simulink model "automata"  (R2020b)
settings: Solver=FixedStepAuto  StartTime=0.0  StopTime=inf  FixedStep=2e-2  RelTol=1e-3
libraries: simulink x3
settings Model: Creator=GoniR  LastModifiedBy=GoniR

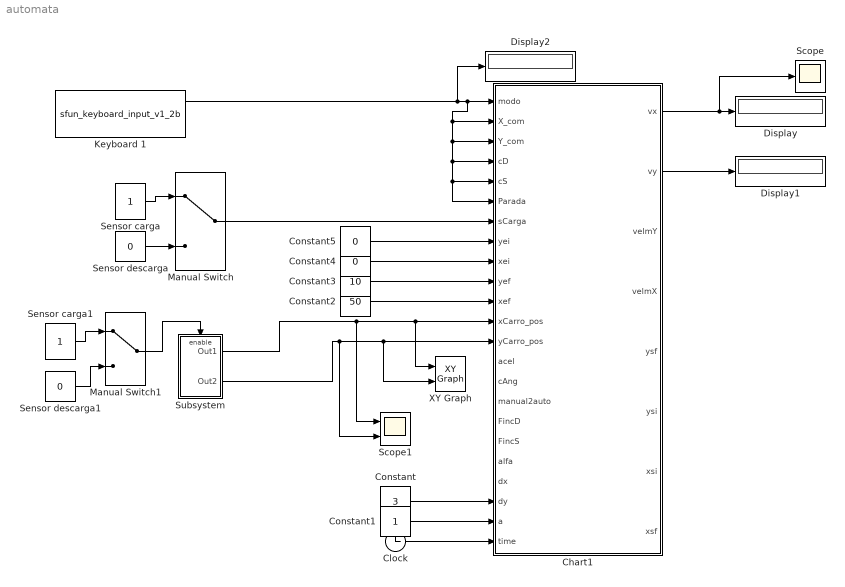
== system automata ==
  Chart1 : Stateflow chart  TreatAsAtomicUnit=on
      settings: PortSchema="{\"entries\":[{\"content\":{\"sides\":[{\"content\":{\"connectorIds\":[\"In5\",\"In1\",\"In2\",\"In12\",\"In13\",\"In18\",\"In14\",\"In9\",\"In10\",\"In4\",\"In11\",\"In16\",\"In22\",\"In23\",\"In15\",\"In3\",\"In17\",\"In19\",\"In7\",\"In8\",\"In6\",\"In21\",\"In20\"]},\"type\":\"ConnectorPlacement.EquallySpacedRectSide\",\"uuid\":\"1e4dd542-1771-4859-b91f-fc1cb250280a\"},{\"content\":{\"connectorIds\":[\"Out1\",\"Out2\",\"Out3\",\"Out4\",\"Out5\",\"Out6\",\"Out7\",\"Out8\"],\"side\":\"RIGHT\"},\"type\":\"ConnectorPlacement.EquallySpacedRectSide\",\"uuid\":\"bb5e6521-c449-4a1c-9147-094c14f63665\"},{\"content\":{\"connectorIds\":[],\"side\":\"TOP\"},\"type\":\"ConnectorPlacement.EquallySpacedRectSide\",\"uuid\":\"54352a45-add1-4eb7-bb1e-2f57d731739f\"},{\"content\":{\"connectorIds\":[],\"side\":\"HIDDEN\"},\"type\":\"ConnectorPlacement.EquallySpacedRectSide\",\"uuid\":\"3e291a91-093a-4ab5-80ab-be4d5a353953\"}]},\"type\":\"ConnectorPlacement.EquallySpacedConnector\",\"uuid\":\"db8c49e8-a9b8-459f-b7fa-0d865c8e3061\"}],\"packageUris\":[\"http://schema.mathworks.com/mf0/Connector/R2020b\"],\"version\":\"1.0\"}"
  Clock : Clock
  Constant : Constant  Value=3
  Constant1 : Constant
  Constant2 : Constant  Value=50
  Constant3 : Constant  Value=10
  Constant4 : Constant  Value=0
  Constant5 : Constant  Value=0
  Display : Display
  Display1 : Display
  Display2 : Display
  Keyboard 1 : M-S-Function  FunctionName=sfun_keyboard_input_v1_2b  mask(Keyboard Input){}
      mask help: Keyboard Input
      mask Display: fprintf('Keyboard');
  Manual Switch : ManualSwitch
  Manual Switch1 : ManualSwitch
  Scope : Scope
  Scope1 : Scope  NumInputPorts=2
  Sensor carga : Constant
  Sensor carga1 : Constant
  Sensor descarga : Constant  Value=0
  Sensor descarga1 : Constant  Value=0
  Subsystem : Subsystem
  XY Graph : simulink/Sinks/XY Graph  xmin=-1  xmax=50  ymin=-1  ymax=30  st=-1
  wires:
  Chart1/1(vx) -> Display/1, Scope/1
  Chart1/2(vy) -> Display1/1
  Sensor carga/1 -> Manual Switch/1
  Sensor descarga/1 -> Manual Switch/2
  Manual Switch/1 -> Chart1/14(sCarga)
  Constant/1 -> Chart1/6(dy)
  Clock/1 -> Chart1/20(time)
  Constant1/1 -> Chart1/21(a)
  Keyboard 1/1 -> Chart1/18(Parada), Chart1/13(cS), Chart1/12(cD), Chart1/2(Y_com), Chart1/1(X_com), Chart1/5(modo), Display2/1
  Constant3/1 -> Chart1/4(yef)
  Constant2/1 -> Chart1/11(xef)
  Constant5/1 -> Chart1/9(yei)
  Constant4/1 -> Chart1/10(xei)
  Subsystem/1(Out1) -> XY Graph/1, Chart1/16(xCarro_pos), Scope1/1
  Subsystem/2(Out2) -> Scope1/2, XY Graph/2, Chart1/22(yCarro_pos)
  Manual Switch1/1 -> Subsystem/Enable
  Sensor descarga1/1 -> Manual Switch1/2
  Sensor carga1/1 -> Manual Switch1/1

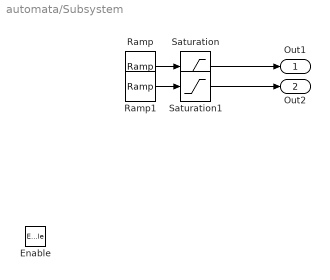
== system automata/Subsystem ==
  Enable : EnablePort
  Ramp : simulink/Sources/Ramp  slope=0.1  start=0  InitialOutput=0
  Ramp1 : simulink/Sources/Ramp  slope=0.1  start=0  InitialOutput=0
  Saturation : Saturate  UpperLimit=50
  Saturation1 : Saturate  UpperLimit=10
  Out1 : Outport
  Out2 : Outport  Port=2
  wires:
  Ramp1/1 -> Saturation1/1
  Saturation/1 -> Out1/1
  Ramp/1 -> Saturation/1
  Saturation1/1 -> Out2/1

== stateflow chart automata/Chart1 ==
  state Nivel1
    state Spreder [parallel]
      settings: executionOrder=1
      state Descargado
        en:
        Scargado=0
      state Cargado
        en:
        Scargado=1
      (default) -> Descargado
      Descargado -> Cargado : [sCarga==1]
      Cargado -> Descargado : [sCarga==0]
    state controlAngulo [parallel]
      settings: executionOrder=2
      state Desactivado
      state Activado
      (default) -> Activado
      Activado -> Desactivado : [cAng==0]
      Desactivado -> Activado : [cAng==1]
    state modoOperacion [parallel]
      settings: executionOrder=3
      state Automatico
        state CicloSimple
          state cargaBarco
            en :
            xsi=xei
            ysi=yei
            xsf=xef
            ysf=yef
            velmX=4
            velmY=1
          state descaragBarco
            en :
            xsi=xei
            ysi=yei
            xsf=xef
            ysf=yef
            velmX=4
            velmY=1
          state standby
          state vueltaMuelle
            en :
            xsi=xei
            ysi=yei
            xsf=xef
            ysf=yef
            velmX=4
            velmY=1
          state idaBarco
            en :
            xsi=xei
            ysi=yei
            xsf=xef
            ysf=yef
            velmX=4
            velmY=1
          Nivel1.modoOperacion.Automatico.CicloSimple.standby -> Nivel1.modoOperacion.Automatico.CicloSimple.cargaBarco [order 1] : [Scargado==1 && xCarro_pos<30 ]
          Nivel1.modoOperacion.Automatico.CicloSimple.standby -> Nivel1.modoOperacion.Automatico.CicloSimple.descaragBarco [order 2] : [Scargado==1 && xCarro_pos<30]
          (default) -> Nivel1.modoOperacion.Automatico.CicloSimple.standby
          Nivel1.modoOperacion.Automatico.CicloSimple.standby -> vueltaMuelle [order 3] : [Scargado==0 && xCarro_pos>30]
          Nivel1.modoOperacion.Automatico.CicloSimple.standby -> idaBarco [order 4] : [Scargado==0 && xCarro_pos<30]
        state standby
        state CicloDoble
          state cargaBarco
            en :
            xsi=xei
            ysi=yei
            xsf=xef
            ysf=yef
            velmX=4
            velmY=1
            error=inf
            du :
            error=Calc_error(xsf,xCarro_pos,ysf,yCarro_pos)
          state standby
          state descaragBarco
            en :
            xsi=xei
            ysi=yei
            xsf=xef
            ysf=yef
            velmX=4
            velmY=1
            error=inf
            du:
            error=Calc_error(xsf,xCarro_pos,ysf,yCarro_pos)
          Nivel1.modoOperacion.Automatico.CicloDoble.standby -> Nivel1.modoOperacion.Automatico.CicloDoble.cargaBarco [order 1] : [xCarro_pos<30]
          (default) -> Nivel1.modoOperacion.Automatico.CicloDoble.standby
          Nivel1.modoOperacion.Automatico.CicloDoble.standby -> Nivel1.modoOperacion.Automatico.CicloDoble.descaragBarco [order 2] : [xCarro_pos>30]
          Nivel1.modoOperacion.Automatico.CicloDoble.descaragBarco -> Nivel1.modoOperacion.Automatico.CicloDoble.cargaBarco : [xCarro_pos<30 && error<1]
          Nivel1.modoOperacion.Automatico.CicloDoble.cargaBarco -> Nivel1.modoOperacion.Automatico.CicloDoble.descaragBarco : [xCarro_pos>30 && error<1]
        Nivel1.modoOperacion.Automatico.standby -> CicloSimple [order 1] : [cS==115]
        CicloSimple -> Nivel1.modoOperacion.Automatico.standby : [Parada==112 || FincS]
        (default) -> Nivel1.modoOperacion.Automatico.standby
        Nivel1.modoOperacion.Automatico.standby -> CicloDoble [order 2] : [cD==100]
        CicloDoble -> Nivel1.modoOperacion.Automatico.standby : [Parada==112 || FincD]
      state modoManual
        en : opManual=1
        vx=0
        vy=0
        time_a=time
        vx_a=0
        du :
        if (X_com == 29 && vx<4)
        vx=acel*(time-time_a)+vx_a
        elseif (X_com == 28 && vx > -4 )
        vx=-acel*(time-time_a)+vx_a
        else
        vx=vx
        end
        du :
        if (Y_com == 31)
        vy=4
        elseif (Y_com==30)
        vy=-4
        else
        vy=0
        end
        time_a=time
        vx_a=vx
      (default) -> modoManual
      modoManual -> Automatico : [modo==97 &&dy>2  ]
      Automatico -> modoManual : [dx<1 && dy<1 && alfa<10 && modo==109]
  (default) -> Nivel1
  data: er function_output; xf function_input; xpos function_input; yf function_input; ypos function_input; X_com input; Y_com input; vx output; opManual local; vy output; manual2auto input; yef input; modo input; dy input; alfa input; dx input; yei input; xei input; xef input; velmY output; velmX output; ysf output; ysi output; xsi output; xsf output; cD input; Scargado local; cS input; sCarga input; cAng input; xCarro_pos input; FincD input; Parada input; FincS input; time input; a input; time_i local; vx_a local; time_a local; yCarro_pos input; error local; acel input
  function er=Calc_error(xf,xpos,yf,ypos):
    | function er=Calc_error(xf,xpos,yf,ypos)
    |     er=((xf-xpos)^2+(yf-ypos)^2)^0.5;
